simulink model "seven_dof_tank_FP_final"  (R2023b)
settings: Solver=VariableStepAuto  StartTime=0.0  StopTime=20  FixedStep=0.000001  RelTol=1e-3
values from neighbouring files (symbols this model uses):
  Be = 100 * ones(7, 1)    [seven_dof_tank_FP_params.m]
  beta = 0.1    [seven_dof_tank_FP_params.m]
  Bh = 2    [seven_dof_tank_FP_params.m]
  Bs = 15    [seven_dof_tank_FP_params.m]
  d = 10    [seven_dof_tank_FP_params.m]
  Dh = 4    [seven_dof_tank_FP_params.m]
  Flp = 5    [seven_dof_tank_FP_params.m]
  Hd = 0.1    [seven_dof_tank_FP_params.m]
  Hm_init = Hd*20    (= 2)    [seven_dof_tank_FP_params.m]
  Hs_init = Hd*20    (= 2)    [seven_dof_tank_FP_params.m]
  Jh = 0    [seven_dof_tank_FP_params.m]
  Ke = 200 * ones(7, 1)    [seven_dof_tank_FP_params.m]
  Ks = 60    [seven_dof_tank_FP_params.m]
  Ph = 2    [seven_dof_tank_FP_params.m]
  q0_m = [0.0167305,-0.762614,-0.0207622,-2.34352,-0.0305686,1.53975,0.753872]'    [seven_dof_tank_FP_params.m]
  q0_s = [0.0167305,-0.762614,-0.0207622,-2.34352,-0.0305686,1.53975,0.753872]'    [seven_dof_tank_FP_params.m]
  tlcAlpha = 0.5    [seven_dof_tank_FP_params.m]
  Ts = 0.001    [seven_dof_tank_FP_params.m]
  xe = [1; 1; 1; 1; 1; 1; 1]    [seven_dof_tank_FP_params.m]
undefined symbols (not defined in the file or in its folder): A, amp_7, Flp1, freq_7, offset_7, phase_7
libraries: simulink x3, cstblocks x1
settings Model: Creator=86180  LastModifiedBy=86180

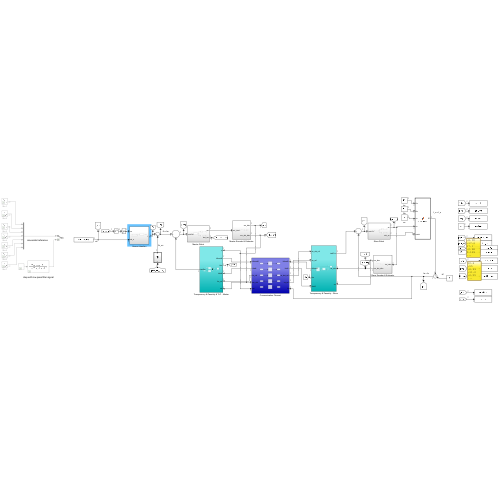
[thumbnail: Simulink's stored preview of the top-level diagram]
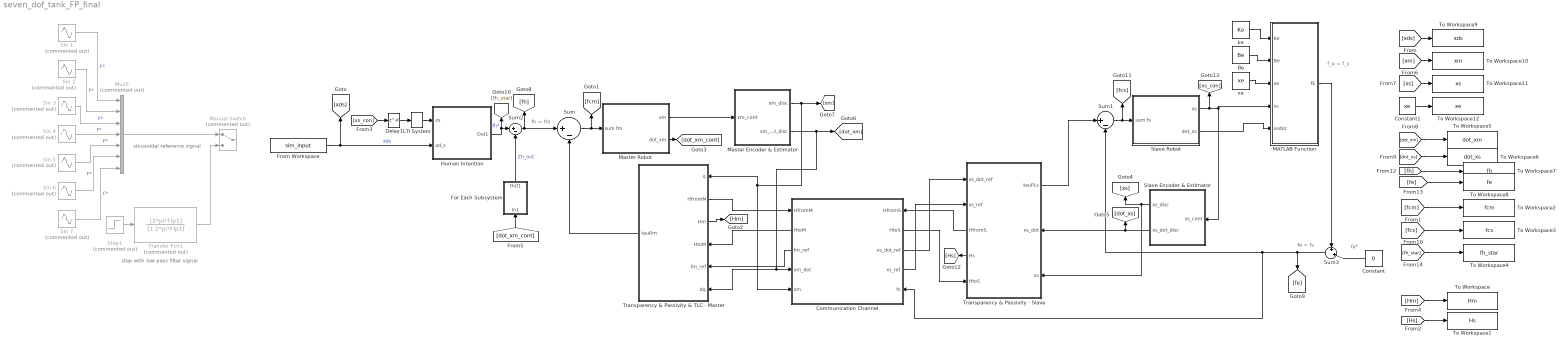
== system seven_dof_tank_FP_final ==
  note: f_e = f_s
  note: fe*
  note: fe = fs
  note: fh = fm
  note: sinusoidal reference signal
  note: step with low pass filter signal
  Be : Constant  Value=Be
  Communication Channel : Subsystem
      settings: PortSchema="{\"entries\":[{\"content\":{\"sides\":[{\"content\":{\"connectorIds\":[\"In1\",\"Out3\",\"Out4\",\"Out5\",\"In2\"]},\"type\":\"ConnectorPlacement.EquallySpacedRectSide\",\"uuid\":\"1c070cf8-9aa7-4f7b-8e2f-2632c2893f69\"},{\"content\":{\"connectorIds\":[\"In3\",\"Out1\",\"Out2\",\"In4\",\"In5\"],\"side\":\"RIGHT\"},\"type\":\"ConnectorPlacement.EquallySpacedRectSide\",\"uuid\":\"32173565-3523-4dfc-9820-763c87098354\"},{\"content\":{\"side\":\"TOP\"},\"type\":\"ConnectorPlacement.EquallySpacedRectSide\",\"uuid\":\"13187df6-bf6f-436e-a2ee-34150977e6a8\"},{\"content\":{\"side\":\"HIDDEN\"},\"type\":\"ConnectorPlacement.EquallySpacedRectSide\",\"uuid\":\"1e5bcdd7-6028-40f7-b524-727817e519ff\"}]},\"type\":\"ConnectorPlacement.EquallySpacedConnector\",\"uuid\":\"c84d0440-83b9-4b92-a10a-1f72bb115b54\"}],\"packageUris\":[\"http://schema.mathworks.com/mf0/Connector/R2020b\"],\"version\":\"1.0\"}"
  Constant : Constant  Value=0
  Constant1 : Constant  Value=xe
  Delay1 : Delay  DelayLength=d  SampleTime=Ts
  For Each Subsystem : Subsystem  TreatAsAtomicUnit=on
  From Workspace : FromWorkspace  VariableName=sim_input  SampleTime=Ts
  Human Intention : Subsystem
  LTI System : cstblocks/LTI System  sys=LTI_Matrix  IC=[]  PadeOrder=0
  MATLAB Function : MATLAB Function  TreatAsAtomicUnit=on
  Manual Switch : ManualSwitch  Commented=on
  Master Encoder & Estimator : Subsystem
  Master Robot : Subsystem
  Mux5 : Mux  Commented=on  Inputs=7
  Sin 1 : Sin  Commented=on  Amplitude=amp_7(1)  Bias=offset_7(1)  Frequency=2*pi*freq_7(1)  Phase=phase_7(1)  SampleTime=0
  Sin 2 : Sin  Commented=on  Amplitude=amp_7(2)  Bias=offset_7(2)  Frequency=2*pi*freq_7(2)  Phase=phase_7(2)  SampleTime=0
  Sin 3 : Sin  Commented=on  Amplitude=amp_7(3)  Bias=offset_7(3)  Frequency=2*pi*freq_7(3)  Phase=phase_7(3)  SampleTime=0
  Sin 4 : Sin  Commented=on  Amplitude=amp_7(4)  Bias=offset_7(4)  Frequency=2*pi*freq_7(4)  Phase=phase_7(4)  SampleTime=0
  Sin 5 : Sin  Commented=on  Amplitude=amp_7(5)  Bias=offset_7(5)  Frequency=2*pi*freq_7(5)  Phase=phase_7(5)  SampleTime=0
  Sin 6 : Sin  Commented=on  Amplitude=amp_7(6)  Bias=offset_7(6)  Frequency=2*pi*freq_7(6)  Phase=phase_7(6)  SampleTime=0
  Sin 7 : Sin  Commented=on  Amplitude=amp_7(7)  Bias=offset_7(7)  Frequency=2*pi*freq_7(7)  Phase=phase_7(7)  SampleTime=0
  Slave Encoder & Estimator : Subsystem
  Slave Robot : Subsystem
  Step1 : Step  Commented=on  Time=0.5  After=A  SampleTime=0
  Sum : Sum  Inputs=|+-
  Sum1 : Sum  Inputs=|+-
  Sum2 : Sum  Inputs=|+-
  Sum3 : Sum  Inputs=+|+|
  To Workspace : ToWorkspace  VariableName=Hm  SaveFormat=Timeseries  SampleTime=-1
  To Workspace1 : ToWorkspace  VariableName=Hs  SaveFormat=Timeseries  SampleTime=-1
  To Workspace10 : ToWorkspace  VariableName=xm  SaveFormat=Timeseries  SampleTime=-1
  To Workspace11 : ToWorkspace  VariableName=xs  SaveFormat=Timeseries  SampleTime=-1
  To Workspace12 : ToWorkspace  VariableName=xe  SaveFormat=Timeseries  SampleTime=-1
  To Workspace2 : ToWorkspace  VariableName=fcm  SaveFormat=Timeseries  SampleTime=-1
  To Workspace3 : ToWorkspace  VariableName=fcs  SaveFormat=Timeseries  SampleTime=-1
  To Workspace4 : ToWorkspace  VariableName=fh_star  SaveFormat=Timeseries  SampleTime=-1
  To Workspace5 : ToWorkspace  VariableName=dot_xm  SaveFormat=Timeseries  SampleTime=-1
  To Workspace6 : ToWorkspace  VariableName=dot_xs  SaveFormat=Timeseries  SampleTime=-1
  To Workspace7 : ToWorkspace  VariableName=fh  SaveFormat=Timeseries  SampleTime=-1
  To Workspace8 : ToWorkspace  VariableName=fe  SaveFormat=Timeseries  SampleTime=-1
  To Workspace9 : ToWorkspace  VariableName=xds  SaveFormat=Timeseries  SampleTime=-1
  Transfer Fcn1 : TransferFcn  Commented=on  Numerator=[2*pi*Flp1]  Denominator=[1 2*pi*Flp1]
  Transparency & Passivity & TLC - Master : Subsystem
      settings: PortSchema="{\"entries\":[{\"content\":{\"sides\":[{\"content\":{\"connectorIds\":[\"In1\",\"Out2\",\"Out3\",\"In2\",\"In3\",\"In4\"]},\"type\":\"ConnectorPlacement.EquallySpacedRectSide\",\"uuid\":\"254acbc8-8c2d-438f-adc1-7e75d47258bf\"},{\"content\":{\"connectorIds\":[\"Out1\"],\"side\":\"RIGHT\"},\"type\":\"ConnectorPlacement.EquallySpacedRectSide\",\"uuid\":\"ebc7579d-fe16-4fae-be7d-b1631322842e\"},{\"content\":{\"side\":\"TOP\"},\"type\":\"ConnectorPlacement.EquallySpacedRectSide\",\"uuid\":\"d0c6f2f9-df1e-40c2-885e-c029821bef96\"}]},\"type\":\"ConnectorPlacement.EquallySpacedConnector\",\"uuid\":\"8dee1f1f-c5e6-463a-a0e9-fbee882b1e3c\"}],\"packageUris\":[\"http://schema.mathworks.com/mf0/Connector/R2020b\"],\"version\":\"1.0\"}"
  Transparency & Passivity - Slave : Subsystem
      settings: PortSchema="{\"entries\":[{\"content\":{\"sides\":[{\"content\":{\"connectorIds\":[\"In1\",\"In2\",\"Out2\",\"Out3\",\"In3\"]},\"type\":\"ConnectorPlacement.EquallySpacedRectSide\",\"uuid\":\"bd42ff73-50dc-42d6-9dfb-d60369543bc9\"},{\"content\":{\"connectorIds\":[\"Out1\",\"In4\",\"In5\"],\"side\":\"RIGHT\"},\"type\":\"ConnectorPlacement.EquallySpacedRectSide\",\"uuid\":\"78e50b8f-eeac-432c-8eb4-27f06d4ce9eb\"},{\"content\":{\"side\":\"TOP\"},\"type\":\"ConnectorPlacement.EquallySpacedRectSide\",\"uuid\":\"9e8e9e88-d3ad-4c46-818b-4ad777acb646\"}]},\"type\":\"ConnectorPlacement.EquallySpacedConnector\",\"uuid\":\"6c4e05d2-6c15-4cd7-9da0-0c4b09a4ecbf\"}],\"packageUris\":[\"http://schema.mathworks.com/mf0/Connector/R2020b\"],\"version\":\"1.0\"}"
  ke : Constant  Value=Ke
  xe : Constant  Value=xe
  wires:
  From Workspace/1 -> [xds], Human Intention/2(xd_s)  "xds"
  For Each Subsystem/1(Out1) -> Sum2/2  "Zh_out"
  Transfer Fcn1/1 -> Manual Switch/2
  Human Intention/1(Out1) -> [fh_star], Sum2/1  "fh*"
  Mux5/1 -> Manual Switch/1
  Step1/1 -> Transfer Fcn1/1
  ke/1 -> MATLAB Function/1(Ke)
  xe/1 -> MATLAB Function/3(xe)
  Slave Robot/1(xs) -> MATLAB Function/4(xs), Slave Encoder & Estimator/1(xs_cont), [xs_con]
  MATLAB Function/1(fE) -> Sum3/1
  Be/1 -> MATLAB Function/2(Be)
  Sum2/1 -> Sum/1, [fh]
  Slave Robot/2(dot_xs) -> MATLAB Function/5(xsdot)
  Sum3/1 -> Communication Channel/2(fs), Sum1/2, [fe]
  Constant/1 -> Sum3/2
  [xds] -> To Workspace9/1
  Sum/1 -> [fcm], Master Robot/1(sum fm)
  [dot_xm_cont] -> For Each Subsystem/1(In1)
  [xm] -> To Workspace10/1
  [dot_xm] -> To Workspace5/1
  Sum1/1 -> [fcs], Slave Robot/1(sum fs)
  [fh] -> To Workspace7/1
  [fe] -> To Workspace8/1
  [fh_star] -> To Workspace4/1
  [fcs] -> To Workspace3/1
  [fcm] -> To Workspace2/1
  [dot_xs] -> To Workspace6/1
  [xs_con] -> Delay1/1
  Master Robot/1(xm) -> Master Encoder & Estimator/1(xm_cont)
  Master Encoder & Estimator/1(xm_disc) -> Communication Channel/5(xm), Transparency & Passivity & TLC - Master/1(q), [xm]
  Master Encoder & Estimator/2(xm_dot_disc) -> Communication Channel/4(xm_dot), Transparency & Passivity & TLC - Master/4(dq), [dot_xm]
  Slave Encoder & Estimator/2(xs_dot_disc) -> Transparency & Passivity - Slave/4(xs_dot), [dot_xs]
  Slave Encoder & Estimator/1(xs_disc) -> Transparency & Passivity - Slave/5(xs), [xs]
  Delay1/1 -> LTI System/1
  LTI System/1 -> Human Intention/1(xs)
  Master Robot/2(dot_xm) -> [dot_xm_cont]
  Transparency & Passivity & TLC - Master/2(HfromM) -> Communication Channel/3(HfromM)
  Transparency & Passivity & TLC - Master/1(tauRm) -> Sum/2
  Communication Channel/1(HtoM) -> Transparency & Passivity & TLC - Master/2(HtoM)
  Communication Channel/2(fm_ref) -> Transparency & Passivity & TLC - Master/3(fm_ref)
  Transparency & Passivity - Slave/2(HfromS) -> Communication Channel/1(HfromS)
  Transparency & Passivity - Slave/1(tauPLs) -> Sum1/1
  Communication Channel/3(HtoS) -> Transparency & Passivity - Slave/3(HtoS)
  Communication Channel/4(xs_dot_ref) -> Transparency & Passivity - Slave/1(xs_dot_ref)
  Communication Channel/5(xs_ref) -> Transparency & Passivity - Slave/2(xs_ref)
  [Hm] -> To Workspace/1
  [Hs] -> To Workspace1/1
  Transparency & Passivity & TLC - Master/3(Hm) -> [Hm]
  Transparency & Passivity - Slave/3(Hs) -> [Hs]
  Sin 1/1 -> Mux5/1  "F*"
  Sin 2/1 -> Mux5/2  "F*"
  Sin 3/1 -> Mux5/3  "F*"
  Sin 4/1 -> Mux5/4  "F*"
  Sin 5/1 -> Mux5/5  "F*"
  Sin 6/1 -> Mux5/6  "F*"
  Sin 7/1 -> Mux5/7  "F*"
  [xs] -> To Workspace11/1
  Constant1/1 -> To Workspace12/1

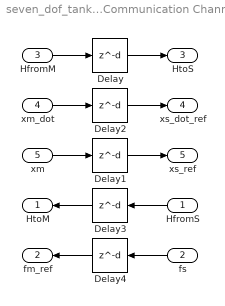
== system seven_dof_tank_FP_final/Communication Channel ==
  HfromS : Inport
  fs : Inport  Port=2
  HfromM : Inport  Port=3
  xm_dot : Inport  Port=4
  xm : Inport  Port=5
  Delay{,1..4} (5 alike) : Delay  DelayLength=d  SampleTime=Ts
  HtoM : Outport
  fm_ref : Outport  Port=2
  HtoS : Outport  Port=3
  xs_dot_ref : Outport  Port=4
  xs_ref : Outport  Port=5
  wires:
  HfromS/1 -> Delay3/1
  xm_dot/1 -> Delay2/1
  fs/1 -> Delay4/1
  Delay4/1 -> fm_ref/1
  xm/1 -> Delay1/1
  Delay1/1 -> xs_ref/1
  Delay2/1 -> xs_dot_ref/1
  HfromM/1 -> Delay/1
  Delay/1 -> HtoS/1
  Delay3/1 -> HtoM/1

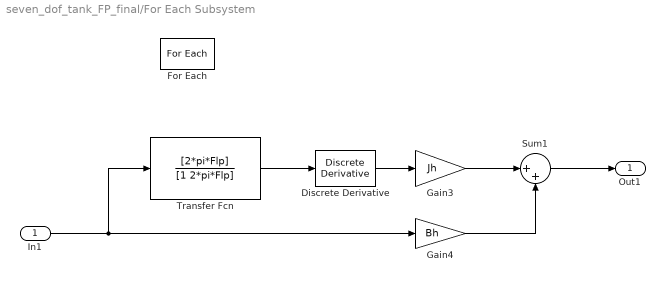
== system seven_dof_tank_FP_final/For Each Subsystem ==
  In1 : Inport  Partition=on  PartitionDimension=1  PartitionWidth=1  PartitionOffset=0
  Discrete Derivative : simulink/Discrete/Discrete Derivative  gainval=1.0  ICPrevScaledInput=0.0  OutMin=[]  OutMax=[]  OutDataType=fixdt(1, 16)  OutScaling=2^-10  DoSatur=off
  For Each : ForEach  DisableCoverage=on
  Gain3 : Gain  Gain=Jh
  Gain4 : Gain  Gain=Bh
  Sum1 : Sum  Inputs=|++
  Transfer Fcn : TransferFcn  Numerator=[2*pi*Flp]  Denominator=[1 2*pi*Flp]
  Out1 : Outport  ConcatenationDimension=1
  wires:
  Gain3/1 -> Sum1/1
  Transfer Fcn/1 -> Discrete Derivative/1
  In1/1 -> Transfer Fcn/1, Gain4/1
  Discrete Derivative/1 -> Gain3/1
  Gain4/1 -> Sum1/2
  Sum1/1 -> Out1/1

== system seven_dof_tank_FP_final/Human Intention ==
  xs : Inport
  xd_s : Inport  Port=2
  For Each Subsystem : Subsystem  TreatAsAtomicUnit=on
  Sum : Sum  Inputs=|-+
  Out1 : Outport
  wires:
  Sum/1 -> For Each Subsystem/1(In1)
  xd_s/1 -> Sum/2
  xs/1 -> Sum/1
  For Each Subsystem/1(Out1) -> Out1/1

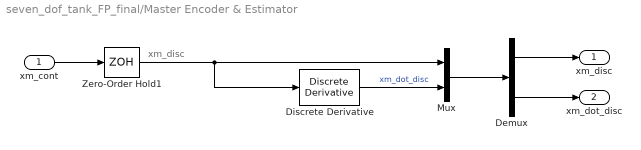
== system seven_dof_tank_FP_final/Master Encoder & Estimator ==
  note: xm_disc
  xm_cont : Inport
  Demux : Demux  Outputs=2
  Discrete Derivative : simulink/Discrete/Discrete Derivative  gainval=1.0  ICPrevScaledInput=0.0  OutMin=[]  OutMax=[]  OutDataType=fixdt(1, 16)  OutScaling=2^-10  DoSatur=off
  Mux : Mux  Inputs=2
  Zero-Order Hold1 : ZeroOrderHold  SampleTime=Ts
  xm_disc : Outport
  xm_dot_disc : Outport  Port=2
  wires:
  Demux/2 -> xm_dot_disc/1
  Discrete Derivative/1 -> Mux/2  "xm_dot_disc"
  Zero-Order Hold1/1 -> Discrete Derivative/1, Mux/1
  xm_cont/1 -> Zero-Order Hold1/1
  Demux/1 -> xm_disc/1
  Mux/1 -> Demux/1

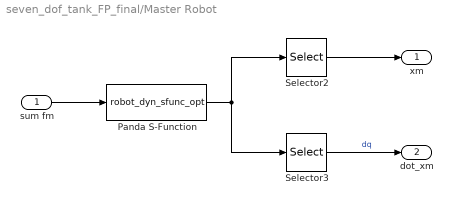
== system seven_dof_tank_FP_final/Master Robot ==
  sum fm : Inport
  Panda S-Function : S-Function  FunctionName=robot_dyn_sfunc_opt  Parameters=q0_m',dq0_m'  SFunctionDeploymentMode=off  EnableBusSupport=off
  Selector2 : Selector  InputPortWidth=14  IndexOptions=Index vector (dialog)  Indices=1:7  OutputSizes=1
  Selector3 : Selector  InputPortWidth=14  IndexOptions=Index vector (dialog)  Indices=8:14  OutputSizes=1
  xm : Outport
  dot_xm : Outport  Port=2
  wires:
  sum fm/1 -> Panda S-Function/1
  Selector3/1 -> dot_xm/1  "dq"
  Panda S-Function/1 -> Selector3/1, Selector2/1
  Selector2/1 -> xm/1

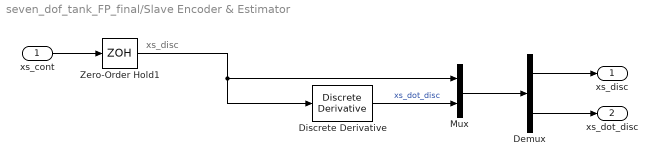
== system seven_dof_tank_FP_final/Slave Encoder & Estimator ==
  note: xs_disc
  xs_cont : Inport
  Demux : Demux  Outputs=2
  Discrete Derivative : simulink/Discrete/Discrete Derivative  gainval=1.0  ICPrevScaledInput=0.0  OutMin=[]  OutMax=[]  OutDataType=fixdt(1, 16)  OutScaling=2^-10  DoSatur=off
  Mux : Mux  Inputs=2
  Zero-Order Hold1 : ZeroOrderHold  SampleTime=Ts
  xs_disc : Outport
  xs_dot_disc : Outport  Port=2
  wires:
  Demux/2 -> xs_dot_disc/1
  Discrete Derivative/1 -> Mux/2  "xs_dot_disc"
  Zero-Order Hold1/1 -> Mux/1, Discrete Derivative/1
  xs_cont/1 -> Zero-Order Hold1/1
  Demux/1 -> xs_disc/1
  Mux/1 -> Demux/1

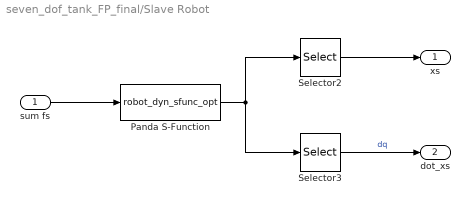
== system seven_dof_tank_FP_final/Slave Robot ==
  sum fs : Inport
  Panda S-Function : S-Function  FunctionName=robot_dyn_sfunc_opt  Parameters=q0_s',dq0_s'  SFunctionDeploymentMode=off  EnableBusSupport=off
  Selector2 : Selector  InputPortWidth=14  IndexOptions=Index vector (dialog)  Indices=1:7  OutputSizes=1
  Selector3 : Selector  InputPortWidth=14  IndexOptions=Index vector (dialog)  Indices=8:14  OutputSizes=1
  xs : Outport
  dot_xs : Outport  Port=2
  wires:
  sum fs/1 -> Panda S-Function/1
  Selector3/1 -> dot_xs/1  "dq"
  Panda S-Function/1 -> Selector3/1, Selector2/1
  Selector2/1 -> xs/1

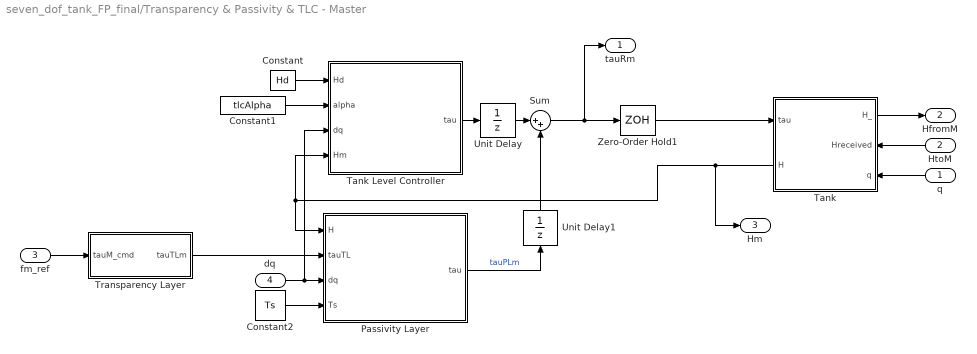
== system seven_dof_tank_FP_final/Transparency & Passivity & TLC - Master ==
  q : Inport
  HtoM : Inport  Port=2
  fm_ref : Inport  Port=3
  dq : Inport  Port=4
  Constant : Constant  Value=Hd
  Constant1 : Constant  Value=tlcAlpha
  Constant2 : Constant  Value=Ts
  Passivity Layer : MATLAB Function  TreatAsAtomicUnit=on
      settings: MinAlgLoopOccurrences=on
  Sum : Sum  Inputs=|++
  Tank : Subsystem  TreatAsAtomicUnit=on
      settings: MinAlgLoopOccurrences=on  PortSchema="{\"entries\":[{\"content\":{\"sides\":[{\"content\":{\"connectorIds\":[\"Out2\",\"In1\",\"In2\"]},\"type\":\"ConnectorPlacement.EquallySpacedRectSide\",\"uuid\":\"482b0a11-f044-49fa-a74d-4dac8b5b787b\"},{\"content\":{\"connectorIds\":[\"In3\",\"Out1\"],\"side\":\"RIGHT\"},\"type\":\"ConnectorPlacement.EquallySpacedRectSide\",\"uuid\":\"b0c369ed-ae40-43d8-b393-bca9f7720d62\"},{\"content\":{\"connectorIds\":[],\"side\":\"TOP\"},\"type\":\"ConnectorPlacement.EquallySpacedRectSide\",\"uuid\":\"ff021616-d6aa-4c0a-874b-a9ebe947c92c\"},{\"content\":{\"connectorIds\":[],\"side\":\"BOTTOM\"},\"type\":\"ConnectorPlacement.EquallySpacedRectSide\",\"uuid\":\"4e18ee96-bca7-41b6-9abb-5b593b41c296\"},{\"content\":{\"connectorIds\":[],\"side\":\"HIDDEN\"},\"type\":\"ConnectorPlacement.EquallySpacedRectSide\",\"uuid\":\"be815b34-35c7-4c6f-8c8b-4a812b3d12e9\"}]},\"type\":\"ConnectorPlacement.EquallySpacedConnector\",\"uuid\":\"78552b8a-5f1c-4815-a807-de98f58b7f2e\"}],\"packageUris\":[\"http://schema.mathworks.com/mf0/Connector/R2020b\"],\"version\":\"1.0\"}"
  Tank Level Controller : MATLAB Function  TreatAsAtomicUnit=on
      settings: MinAlgLoopOccurrences=on
  Transparency Layer : Subsystem
  Unit Delay : UnitDelay  SampleTime=-1  HasFrameUpgradeWarning=on
  Unit Delay1 : UnitDelay  SampleTime=-1  HasFrameUpgradeWarning=on
  Zero-Order Hold1 : ZeroOrderHold  SampleTime=Ts
  tauRm : Outport
  HfromM : Outport  Port=2
  Hm : Outport  Port=3
  wires:
  Tank Level Controller/1(tau) -> Unit Delay/1
  Passivity Layer/1(tau) -> Unit Delay1/1  "tauPLm"
  Zero-Order Hold1/1 -> Tank/3(tau)
  Tank/1(H) -> Hm/1, Passivity Layer/1(H), Tank Level Controller/4(Hm)
  fm_ref/1 -> Transparency Layer/1(tauM_cmd)
  Transparency Layer/1(tauTLm) -> Passivity Layer/2(tauTL)
  dq/1 -> Tank Level Controller/3(dq), Passivity Layer/3(dq)
  Constant2/1 -> Passivity Layer/4(Ts)
  Tank/2(H_) -> HfromM/1
  Constant/1 -> Tank Level Controller/1(Hd)
  Constant1/1 -> Tank Level Controller/2(alpha)
  Sum/1 -> tauRm/1, Zero-Order Hold1/1
  q/1 -> Tank/2(q)
  HtoM/1 -> Tank/1(Hreceived)
  Unit Delay/1 -> Sum/1
  Unit Delay1/1 -> Sum/2

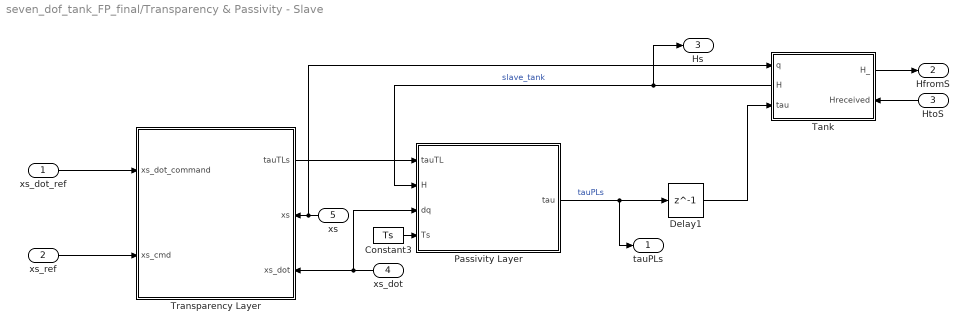
== system seven_dof_tank_FP_final/Transparency & Passivity - Slave ==
  xs_dot_ref : Inport
  xs_ref : Inport  Port=2
  HtoS : Inport  Port=3
  xs_dot : Inport  Port=4
  xs : Inport  Port=5
  Constant3 : Constant  Value=Ts
  Delay1 : Delay  DelayLength=1  SampleTime=Ts
  Passivity Layer : MATLAB Function  TreatAsAtomicUnit=on
  Tank : Subsystem
      settings: PortSchema="{\"entries\":[{\"content\":{\"sides\":[{\"content\":{\"connectorIds\":[\"In1\",\"Out2\",\"In2\"]},\"type\":\"ConnectorPlacement.EquallySpacedRectSide\",\"uuid\":\"482b0a11-f044-49fa-a74d-4dac8b5b787b\"},{\"content\":{\"connectorIds\":[\"Out1\",\"In3\"],\"side\":\"RIGHT\"},\"type\":\"ConnectorPlacement.EquallySpacedRectSide\",\"uuid\":\"b0c369ed-ae40-43d8-b393-bca9f7720d62\"},{\"content\":{\"connectorIds\":[],\"side\":\"TOP\"},\"type\":\"ConnectorPlacement.EquallySpacedRectSide\",\"uuid\":\"ff021616-d6aa-4c0a-874b-a9ebe947c92c\"},{\"content\":{\"connectorIds\":[],\"side\":\"BOTTOM\"},\"type\":\"ConnectorPlacement.EquallySpacedRectSide\",\"uuid\":\"4e18ee96-bca7-41b6-9abb-5b593b41c296\"},{\"content\":{\"connectorIds\":[],\"side\":\"HIDDEN\"},\"type\":\"ConnectorPlacement.EquallySpacedRectSide\",\"uuid\":\"be815b34-35c7-4c6f-8c8b-4a812b3d12e9\"}]},\"type\":\"ConnectorPlacement.EquallySpacedConnector\",\"uuid\":\"78552b8a-5f1c-4815-a807-de98f58b7f2e\"}],\"packageUris\":[\"http://schema.mathworks.com/mf0/Connector/R2020b\"],\"version\":\"1.0\"}"
  Transparency Layer : Subsystem
      settings: PortSchema="{\"entries\":[{\"content\":{\"sides\":[{\"content\":{\"connectorIds\":[\"In1\",\"In2\"]},\"type\":\"ConnectorPlacement.EquallySpacedRectSide\",\"uuid\":\"c8f256d1-8287-4bc6-9264-40c0684f6acd\"},{\"content\":{\"connectorIds\":[\"Out1\",\"In3\",\"In4\"],\"side\":\"RIGHT\"},\"type\":\"ConnectorPlacement.EquallySpacedRectSide\",\"uuid\":\"cb9f571e-93fc-426e-a4f2-aa96ae3bd6b3\"},{\"content\":{\"side\":\"TOP\"},\"type\":\"ConnectorPlacement.EquallySpacedRectSide\",\"uuid\":\"b9b91304-f20e-4a66-aa64-b99c686ee85a\"},{\"content\":{\"side\":\"HIDDEN\"},\"type\":\"ConnectorPlacement.EquallySpacedRectSide\",\"uuid\":\"c3abcf5a-e3b9-4b9a-a4b1-68c5725be1f4\"}]},\"type\":\"ConnectorPlacement.EquallySpacedConnector\",\"uuid\":\"83907002-acbd-4948-aeba-a43201e13c19\"}],\"packageUris\":[\"http://schema.mathworks.com/mf0/Connector/R2020b\"],\"version\":\"1.0\"}"
  tauPLs : Outport
  HfromS : Outport  Port=2
  Hs : Outport  Port=3
  wires:
  xs_dot_ref/1 -> Transparency Layer/1(xs_dot_command)
  xs_ref/1 -> Transparency Layer/2(xs_cmd)
  Transparency Layer/1(tauTLs) -> Passivity Layer/1(tauTL)
  xs/1 -> Tank/1(q), Transparency Layer/3(xs)
  Constant3/1 -> Passivity Layer/4(Ts)
  xs_dot/1 -> Passivity Layer/3(dq), Transparency Layer/4(xs_dot)
  Tank/2(H) -> Hs/1, Passivity Layer/2(H)  "slave_tank"
  Passivity Layer/1(tau) -> tauPLs/1, Delay1/1  "tauPLs"
  Delay1/1 -> Tank/2(tau)
  Tank/1(H_) -> HfromS/1
  HtoS/1 -> Tank/3(Hreceived)

== system seven_dof_tank_FP_final/Human Intention/For Each Subsystem ==
  In1 : Inport  Partition=on  PartitionDimension=1  PartitionWidth=1  PartitionOffset=0
  For Each : ForEach  DisableCoverage=on
  Transfer Fcn : TransferFcn  Numerator=[Dh Ph]  Denominator=[1 0]
  Out1 : Outport  ConcatenationDimension=1
  wires:
  In1/1 -> Transfer Fcn/1
  Transfer Fcn/1 -> Out1/1

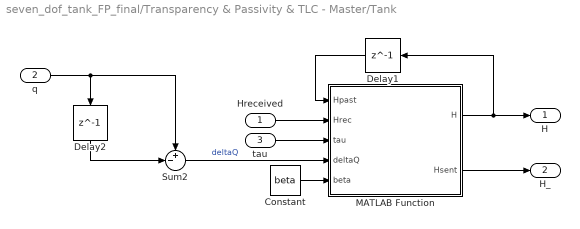
== system seven_dof_tank_FP_final/Transparency & Passivity & TLC - Master/Tank ==
  Hreceived : Inport
  q : Inport  Port=2
  tau : Inport  Port=3
  Constant : Constant  Value=beta
  Delay1 : Delay  DelayLength=1  InitialCondition=Hm_init  SampleTime=Ts
  Delay2 : Delay  DelayLength=1  SampleTime=Ts
  MATLAB Function : MATLAB Function  TreatAsAtomicUnit=on
  Sum2 : Sum  Inputs=+-|
  H : Outport
  H_ : Outport  Port=2
  wires:
  Delay2/1 -> Sum2/2
  q/1 -> Sum2/1, Delay2/1
  MATLAB Function/2(Hsent) -> H_/1
  Constant/1 -> MATLAB Function/5(beta)
  Sum2/1 -> MATLAB Function/4(deltaQ)  "deltaQ"
  Hreceived/1 -> MATLAB Function/2(Hrec)
  tau/1 -> MATLAB Function/3(tau)
  MATLAB Function/1(H) -> Delay1/1, H/1
  Delay1/1 -> MATLAB Function/1(Hpast)

== system seven_dof_tank_FP_final/Transparency & Passivity & TLC - Master/Transparency Layer ==
  tauM_cmd : Inport
  tauTLm : Outport
  wires:
  tauM_cmd/1 -> tauTLm/1

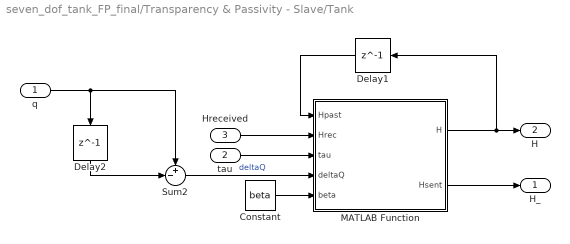
== system seven_dof_tank_FP_final/Transparency & Passivity - Slave/Tank ==
  q : Inport
  tau : Inport  Port=2
  Hreceived : Inport  Port=3
  Constant : Constant  Value=beta
  Delay1 : Delay  DelayLength=1  InitialCondition=Hs_init  SampleTime=Ts
  Delay2 : Delay  DelayLength=1  SampleTime=Ts
  MATLAB Function : MATLAB Function  TreatAsAtomicUnit=on
  Sum2 : Sum  Inputs=+-|
  H_ : Outport
  H : Outport  Port=2
  wires:
  Delay2/1 -> Sum2/2
  q/1 -> Sum2/1, Delay2/1
  MATLAB Function/2(Hsent) -> H_/1
  Constant/1 -> MATLAB Function/5(beta)
  Sum2/1 -> MATLAB Function/4(deltaQ)  "deltaQ"
  Hreceived/1 -> MATLAB Function/2(Hrec)
  tau/1 -> MATLAB Function/3(tau)
  MATLAB Function/1(H) -> Delay1/1, H/1
  Delay1/1 -> MATLAB Function/1(Hpast)

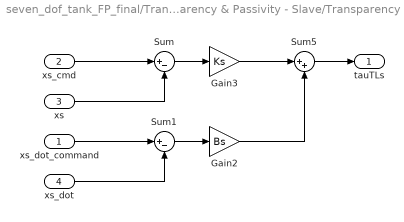
== system seven_dof_tank_FP_final/Transparency & Passivity - Slave/Transparency Layer ==
  xs_dot_command : Inport
  xs_cmd : Inport  Port=2
  xs : Inport  Port=3
  xs_dot : Inport  Port=4
  Gain2 : Gain  Gain=Bs
  Gain3 : Gain  Gain=Ks
  Sum : Sum  Inputs=|+-
  Sum1 : Sum  Inputs=|+-
  Sum5 : Sum  Inputs=|++
  tauTLs : Outport
  wires:
  Sum5/1 -> tauTLs/1
  xs/1 -> Sum/2
  xs_dot/1 -> Sum1/2
  xs_cmd/1 -> Sum/1
  xs_dot_command/1 -> Sum1/1
  Sum/1 -> Gain3/1
  Sum1/1 -> Gain2/1
  Gain3/1 -> Sum5/1
  Gain2/1 -> Sum5/2

== matlab function seven_dof_tank_FP_final/Transparency & Passivity & TLC - Master/Tank/MATLAB Function ==
  data: Hpast input; H output; Hrec input; tau input; deltaQ input; beta input; Hsent output
function [H, Hsent] = tank(Hpast, Hrec, tau, deltaQ, beta)
    % 各关节的能量消耗
    Hused = tau .* deltaQ; % .* 表示逐元素相乘
    % 更新总能量
    H = Hpast + Hrec - Hused; 
    % 计算传输能量
    Hsent = H .* beta; 
    % 更新H
    H = H - Hsent; 
end

== matlab function seven_dof_tank_FP_final/MATLAB Function ==
  data: Ke input; fE output; Be input; xe input; xs input; xsdot input
function fE = environment(Ke, Be, xe, xs, xsdot)
% 支持 7DoF 环境交互力计算
% 输入:
% - Ke: 刚度向量 (7×1)
% - Be: 阻尼系数向量 (7×1)
% - xe: 环境位置向量 (7×1)
% - xs: 从机器人当前位置向量 (7×1)
% - xsdot: 从机器人速度向量 (7×1)
% 输出:
% - fE: 环境交互力向量 (7×1)

% 初始化交互力
fE = zeros(7, 1);

% 对每个关节分别计算
for i = 1:7
    if xs(i) > xe(i)
        fE(i) = Ke(i) * (xs(i) - xe(i)) + Be(i) * max(xsdot(i), 0);
    else
        fE(i) = 0;
    end
end

end

== matlab function seven_dof_tank_FP_final/Transparency & Passivity & TLC - Master/Tank Level Controller ==
  data: Hd input; alpha input; dq input; tau output; Hm input
function tau = TLC(Hd, alpha, dq, Hm)
% TLC - 计算 7 自由度系统的力矩反馈控制
%
% 输入:
%   Hd    - 目标罐能量 (标量, 共用值)
%   alpha - 控制系数 (标量, 共用值)
%   dq    - 关节速度 (7×1 向量)
%   Hm    - 当前罐能量 (7×1 向量)
%
% 输出:
%   tau   - 输出控制力矩 (7×1 向量)

% 初始化 tau
tau = zeros(7, 1);

% 对每个自由度单独计算 tau
for i = 1:7
    if Hd <= Hm(i)
        d = 0;
    else
        d = alpha * (Hd - Hm(i));  % 使用共用的标量 Hd 和 alpha
    end
    tau(i) = -d * dq(i);  % 每个自由度独立计算 tau
end

== matlab function seven_dof_tank_FP_final/Transparency & Passivity - Slave/Passivity Layer ==
  data: tauTL input; H input; tau output; dq input; Ts input
function tau = tauPL(tauTL, H, dq,Ts)
% Slide 23 (改为支持7DoF)
% 输入:
% - H: 罐能量 (7×1向量, 每个关节的能量)
% - tauTL: 输入力矩限制 (7×1向量)
% - dq: 关节速度 (7×1向量)
% - Ts: 仿真步长 (标量)
% 输出:
% - tau: 输出限制后的关节力矩 (7×1向量)

% 初始化 tauMax1 和 tauMax2
tauMax1 = zeros(7, 1);
tauMax2 = zeros(7, 1);

% 循环每个关节计算
for i = 1:7
    % tauMax1 计算
    if H(i) <= 0
        tauMax1(i) = 0;
    else
        tauMax1(i) = tauTL(i);
    end

    % tauMax2 计算
    tauMax2(i) = H(i) / (dq(i) * Ts);
end

% 输出限制力矩 tau
tau = sign(tauTL) .* min(abs(tauMax1), abs(tauMax2));

end

== matlab function seven_dof_tank_FP_final/Transparency & Passivity & TLC - Master/Passivity Layer ==
  data: H input; tauTL input; dq input; Ts input; tau output
function tau = PL(H, tauTL, dq, Ts)
% Slide 23 (改为支持7DoF)
% 输入:
% - H: 罐能量 (7×1向量, 每个关节的能量)
% - tauTL: 输入力矩限制 (7×1向量)
% - dq: 关节速度 (7×1向量)
% - Ts: 仿真步长 (标量)
% 输出:
% - tau: 输出限制后的关节力矩 (7×1向量)

% 初始化 tauMax1 和 tauMax2
tauMax1 = zeros(7, 1);
tauMax2 = zeros(7, 1);

% 循环每个关节计算
for i = 1:7
    % tauMax1 计算
    if H(i) <= 0
        tauMax1(i) = 0;
    else
        tauMax1(i) = tauTL(i);
    end

    % tauMax2 计算
    tauMax2(i) = H(i) / (dq(i) * Ts);
end

% 输出限制力矩 tau
tau = sign(tauTL) .* min(abs(tauMax1), abs(tauMax2));

end

== matlab function seven_dof_tank_FP_final/Transparency & Passivity - Slave/Tank/MATLAB Function ==
  data: Hpast input; H output; Hrec input; tau input; deltaQ input; beta input; Hsent output
function [H, Hsent] = tank(Hpast, Hrec, tau, deltaQ, beta)
    % 各关节的能量消耗
    Hused = tau .* deltaQ; % .* 表示逐元素相乘
    % 更新总能量
    H = Hpast + Hrec - Hused; 
    % 计算传输能量
    Hsent = H .* beta; 
    % 更新H
    H = H - Hsent; 
end
